simulink model "motor_ctrl_reference"  (R2020b)
settings: Solver=VariableStepAuto  StartTime=0.0  StopTime=1  RelTol=1e-3
InitFcn:
  | Rs=0.43;
  | 
  | Lls=0.002
  | 
  | Rr=0.816;
  | 
  | Llr=0.002
  | 
  | Lm=0.6931;
  | 
  | 
  | J=0.085;
  | np=2;
  | 
  | Ts=1e-5;
  | 
  | Udc=400*sqrt(3)
  | Tpwm = 1e-4;
  | 
  | 
  | 
  | Ls = 1.5*Lm+Lls
  | Lr = 1.5*Lm+Llr
  | Tr = Lr/Rr;
  | sigma = (Ls*Lr-Lm*Lm)/Ls/Lr;
libraries: powerlib x12, simulink x2
settings Model: Creator=messer  LastModifiedBy=messer

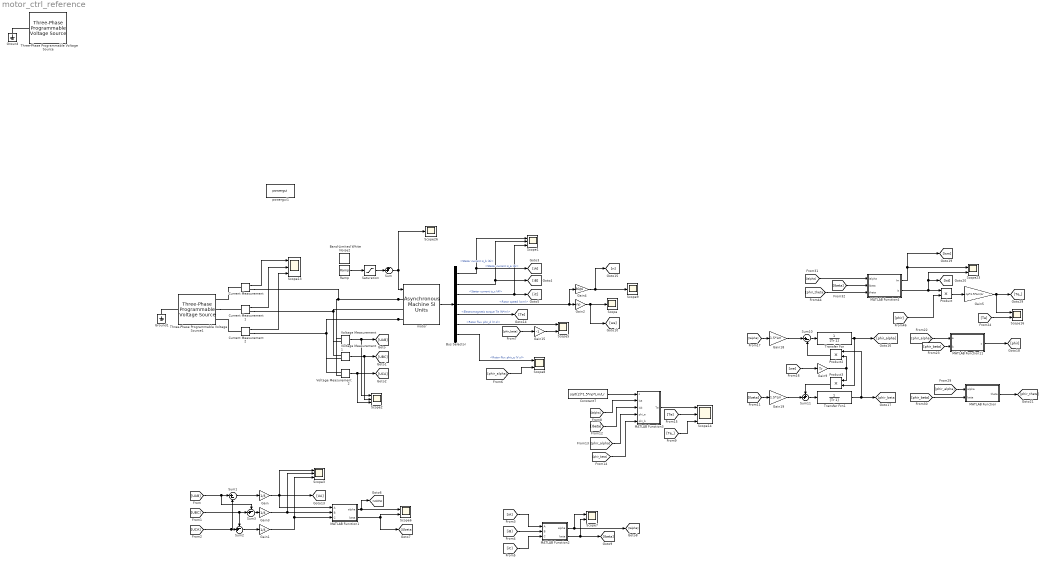
== system motor_ctrl_reference ==
  Band-Limited White Noise2 : simulink/Sources/Band-Limited White Noise  Cov=[0.0001]  Ts=1e-4  seed=[130341]
  Bus Selector : BusSelector  OutputSignals=Stator measurements.Stator current is_a (A),Stator measurements.Stator current is_b (A),Stator measurements.Stator current is_c (A),Mechanical.Rotor speed (wm),Mechanical.Electromagnetic torque Te (N*m),Rotor measurements.Rotor flux phir_d (V s),Rotor measurements.Rotor flux phir_q (V s)
  Constant7 : Constant  Value=sqrt(2)*1.5*np*Lm/Lr
  Current Measurement : powerlib/Measurements/Current Measurement  PhasorSimulation=off  OutputType=Complex  PSBequivalent=0
  Current Measurement1 : powerlib/Measurements/Current Measurement  PhasorSimulation=off  OutputType=Complex  PSBequivalent=0
  Current Measurement2 : powerlib/Measurements/Current Measurement  PhasorSimulation=off  OutputType=Complex  PSBequivalent=0
  Gain : Gain  Gain=1/3
  Gain1 : Gain  Gain=1/3
  Gain15 : Gain  Gain=-1
  Gain18 : Gain  Gain=1.5*Lm
  Gain19 : Gain  Gain=1.5*Lm
  Gain2 : Gain  Gain=np
  Gain3 : Gain  Gain=1/3
  Gain4 : Gain  Gain=30/pi
  Gain5 : Gain  Gain=np*1.5*Lm/Lr
  Gain9 : Gain  Gain=Tr
  Ground : powerlib/Elements/Ground  LConnTagsString=a
  Ground1 : powerlib/Elements/Ground  LConnTagsString=a
  MATLAB Function : MATLAB Function  TreatAsAtomicUnit=on
  MATLAB Function1 : MATLAB Function  TreatAsAtomicUnit=on
  MATLAB Function11 : MATLAB Function  TreatAsAtomicUnit=on
  MATLAB Function2 : MATLAB Function  TreatAsAtomicUnit=on
  MATLAB Function3 : MATLAB Function  TreatAsAtomicUnit=on
  MATLAB Function4 : MATLAB Function  TreatAsAtomicUnit=on
  Product : Product
  Product2 : Product
  Product3 : Product
  Ramp : simulink/Sources/Ramp  slope=100  start=0.25  InitialOutput=5
  Saturation : Saturate  UpperLimit=20  LowerLimit=0
  Scope : Scope
  Scope{1..3,13..14} (5 alike) : Scope  NumInputPorts=3
  Scope{5..8,16,23} (6 alike) : Scope  NumInputPorts=2
  Scope26 : Scope
  Scope9 : Scope
  Sum : Sum  Inputs=++|
  Sum1 : Sum  Inputs=|+-
  Sum10 : Sum  Inputs=|+-
  Sum11 : Sum  Inputs=++|
  Sum2 : Sum  Inputs=-+|
  Sum3 : Sum  Inputs=-+|
  Three-Phase Programmable Voltage Source : powerlib/Electrical Sources/Three-Phase Programmable Voltage Source  PositiveSequence="[380/sqrt(2)  0 50]"  VariationEntity=None  VariationType=Table of time-amplitude pairs  VariationTypeAlt=Step  VariationStep=0.5  VariationRate=10  VariationMagnitude=0.3  VariationFrequency=2  VariationTiming=[1 2]  VariationPhaseA=off  Amplitudes=[1 0.8 1.2 1.0]  TimeValues=[0 0.1 0.15 0.2]  HarmonicGeneration=off  HarmonicA=[3 0.2 -25 0]  HarmonicB=[2 0.15 35 2]  Timing="[0.05  3]"  BusType=swing  Pref=0  Qref=0  Qmin=-inf  Qmax=inf
  Three-Phase Programmable Voltage Source1 : powerlib/Electrical Sources/Three-Phase Programmable Voltage Source  PositiveSequence="[400*sqrt(3/2)  0 120]"  VariationEntity=None  VariationType=Table of time-amplitude pairs  VariationTypeAlt=Step  VariationStep=0.5  VariationRate=10  VariationMagnitude=0.3  VariationFrequency=2  VariationTiming=[1 2]  VariationPhaseA=off  Amplitudes=[1 0.8 1.2 1.0]  TimeValues=[0 0.1 0.15 0.2]  HarmonicGeneration=off  HarmonicA=[3 0.2 -25 0]  HarmonicB=[2 0.15 35 2]  Timing="[0.05  3]"  BusType=swing  Pref=0  Qref=0  Qmin=-inf  Qmax=inf
  Transfer Fcn : TransferFcn  Denominator=[Tr 1]
  Transfer Fcn1 : TransferFcn  Denominator=[Tr 1]
  Voltage Measurement : powerlib/Measurements/Voltage Measurement  PhasorSimulation=off  OutputType=Complex  PSBequivalent=0
  Voltage Measurement1 : powerlib/Measurements/Voltage Measurement  PhasorSimulation=off  OutputType=Complex  PSBequivalent=0
  Voltage Measurement2 : powerlib/Measurements/Voltage Measurement  PhasorSimulation=off  OutputType=Complex  PSBequivalent=0
  motor : powerlib/Machines/Asynchronous Machine SI Units  RotorType=Squirrel-cage  PresetModel=No  MechanicalLoad=Torque Tm  ShowDetailedParameters=on  ReferenceFrame=Stationary  Units=SI  MeasurementBus=off  NominalParameters=[562000 2750 135]  Stator=[Rs Lls]  Rotor=[Rr Llr]  Cage1=[0.4155 0.002066]  Cage2=[0.4168 0.0003495]  Lm=Lm  Mechanical=[J 0 np]  PolePairs=2  InitialConditions=[1 0 0 0 0 0 0 0]  SimulateSaturation=off  Saturation=[14.03593122, 27.81365428, 53.79336849, 72.68890987, 97.98006896, 148.6815601, 215.7428561, 302.9841135, 428.7778367 ; 230, 322, 414, 460, 506, 552, 598, 644, 690]  LoadFlowParameters=1492000  TsPowergui=0  TsBlock=-1  IterativeModel=Trapezoidal non iterative  IterativeDiscreteModel=Trapezoidal non iterative  Pmec=1.492e+006
  powergui1 : powerlib/powergui  Priority=1  SimulationMode=Discrete  SampleTime=2e-6  frequency=60  Iterations=50  frequencyindice=120  Pbase=100e6  ErrMax=1e-4  UnitsV=kV  UnitsW=MW  buscounter=0  FunctionMessages=off  echomessages=off  EnableUseOfTLC=off  CurrentSourceSwitches=off  DisableSnubberDevices=off  DisableRonSwitches=off  DisableVfSwitches=off  DisplayEquations=off  AutomaticDiscreteSolvers=off  SolverType=Tustin/Backward Euler (TBE)  Interpol=off  ExternalGateDelay=off  methode=off  Ts=100  x0status=blocks  SPID=on  SwTol=0  HookPort=off  NonlinearTolerance=1e-4  nMaxIteration=100  ContinueOnMaxIteration=off  RestoreLinks=warning  ResistiveCurrentMeasurement=off  Frange=[0:2:500]  Ylog=off  Xlog=on  ShowGrid=off  save=off  variable=ZData  structure=0  ZoomFFT=off  StartTime=0.0  cycles=1  DisplayStyle=1  fundamental=60  FreqAxis=off  MaxFrequency=1000  frequencyindicesteady=1  RmsSteady=1  display=off
  wires:
  Transfer Fcn/1 -> Product3/2, [phir_alpha]
  Sum10/1 -> Transfer Fcn/1
  MATLAB Function/1(theta) -> [phir_theta]
  Gain9/1 -> Product3/1, Product2/2
  Transfer Fcn1/1 -> Product2/1, [phir_beta]
  Sum11/1 -> Transfer Fcn1/1
  [Ialpha] -> Gain18/1
  [UBC] -> Sum2/1, Sum3/2
  [Ibeta] -> Gain19/1
  Product3/1 -> Sum11/1
  Product2/1 -> Sum10/2
  Gain1/1 -> MATLAB Function1/3(C), Scope3/3
  Gain19/1 -> Sum11/2
  motor/1 -> Bus Selector/1
  MATLAB Function4/1(Im) -> [Ism], Scope23/1
  MATLAB Function11/1(y) -> [phir]
  [we] -> Gain9/1
  [iB] -> MATLAB Function2/2(B)
  Product/1 -> Gain5/1
  [phir_beta] -> MATLAB Function3/5(phi_b)
  [phir_beta] -> MATLAB Function/2(beta)
  Gain18/1 -> Sum10/1
  [phir_theta] -> MATLAB Function4/3(theta)
  MATLAB Function1/2(beta) -> [Ubeta], Scope6/2
  [phir] -> Product/2
  Gain2/1 -> [we], Scope/1
  [Te] -> Scope16/2
  Bus Selector/5 -> [Te]  "<Electromagnetic torque Te (N*m)>"
  [phir_beta] -> Gain15/1
  Gain15/1 -> Scope5/2
  [phir_alpha] -> Scope8/2
  [iA] -> MATLAB Function2/1(A)
  Gain5/1 -> [Te_], Scope16/1
  Current Measurement2/1 -> Scope13/3
  Bus Selector/4 -> Gain4/1, Gain2/1  "<Rotor speed (wm)>"
  [UCA] -> Sum1/2, Sum2/2
  Ramp/1 -> Saturation/1
  Current Measurement1/1 -> Scope13/2
  MATLAB Function2/1(alpha) -> Scope7/1, [Ialpha]
  [Ialpha] -> MATLAB Function4/1(Ialpha)
  Current Measurement/1 -> Scope13/1
  MATLAB Function4/2(It) -> Scope23/2, [Ist], Product/1
  [Ibeta] -> MATLAB Function4/2(Ibeta)
  [phir_beta] -> MATLAB Function11/2(b)
  [phir_alpha] -> MATLAB Function11/1(a)
  MATLAB Function3/1(Te) -> Scope14/1
  Bus Selector/1 -> [iA], Scope1/1  "<Stator current is_a (A)>"
  [phir_alpha] -> MATLAB Function3/4(phi_a)
  Sum/1 -> Scope26/1, motor/1
  Voltage Measurement2/1 -> [UCA], Scope2/3
  Bus Selector/3 -> Scope1/3, [iC]  "<Stator current is_c (A)>"
  Bus Selector/6 -> Scope5/1  "<Rotor flux phir_d (V s)>"
  Gain4/1 -> [n], Scope9/1
  Gain/1 -> MATLAB Function1/1(A), [UA], Scope3/1
  Constant7/1 -> MATLAB Function3/1(c)
  MATLAB Function2/2(beta) -> [Ibeta], Scope7/2
  MATLAB Function1/1(alpha) -> [Ualpha], Scope6/1
  [phir_alpha] -> MATLAB Function/1(alpha)
  [Ialpha] -> MATLAB Function3/2(isa)
  [UAB] -> Sum3/1, Sum1/1
  [Te_] -> Scope14/3
  [Te] -> Scope14/2
  Bus Selector/2 -> Scope1/2, [iB]  "<Stator current is_b (A)>"
  [Ibeta] -> MATLAB Function3/3(isb)
  Sum3/1 -> Gain3/1
  Sum1/1 -> Gain/1
  [iC] -> MATLAB Function2/3(C)
  Saturation/1 -> Sum/2
  Voltage Measurement1/1 -> [UBC], Scope2/2
  Sum2/1 -> Gain1/1
  Bus Selector/7 -> Scope8/1  "<Rotor flux phir_q (V s)>"
  Gain3/1 -> MATLAB Function1/2(B), Scope3/2
  Voltage Measurement/1 -> Scope2/1, [UAB]
  connections:
  Ground/LConn1 -- Three-Phase Programmable Voltage Source/LConn1
  motor/LConn1 -- Voltage Measurement/LConn1 -- Voltage Measurement2/LConn2 -- Current Measurement/RConn1
  Current Measurement1/RConn1 -- Voltage Measurement1/LConn1 -- Voltage Measurement/LConn2 -- motor/LConn2
  motor/LConn3 -- Current Measurement2/RConn1 -- Voltage Measurement2/LConn1 -- Voltage Measurement1/LConn2
  Ground1/LConn1 -- Three-Phase Programmable Voltage Source1/LConn1
  Three-Phase Programmable Voltage Source1/RConn2 -- Current Measurement1/LConn1
  Current Measurement/LConn1 -- Three-Phase Programmable Voltage Source1/RConn1
  Current Measurement2/LConn1 -- Three-Phase Programmable Voltage Source1/RConn3

== matlab function motor_ctrl_reference/MATLAB Function1 ==
  data: A input; alpha output; B input; C input; beta output
function [alpha, beta] = fcn(A, B, C)
k = 2/ 3;
alpha = k * (A - 0.5*B - 0.5*C);
beta = k * sqrt(3) / 2 * (B - C);

== matlab function motor_ctrl_reference/MATLAB Function2 ==
  data: A input; alpha output; B input; C input; beta output
function [alpha, beta] = fcn(A, B, C)
k = 2/ 3;
alpha = k * (A - 0.5*B - 0.5*C);
beta = k * sqrt(3) / 2 * (B - C);

== matlab function motor_ctrl_reference/MATLAB Function3 ==
  data: c input; Te output; isa input; isb input; phi_a input; phi_b input
function Te = fcn(c, isa, isb, phi_a, phi_b)
Te = c *( isb * phi_a - isa * phi_b);

== matlab function motor_ctrl_reference/MATLAB Function4 ==
  data: Im output; Ialpha input; Ibeta input; theta input; It output
function [Im, It] = fcn(Ialpha, Ibeta, theta)

Im = Ialpha * cos(theta) + Ibeta * sin(theta);
It = -Ialpha * sin(theta) + Ibeta * cos(theta);

== matlab function motor_ctrl_reference/MATLAB Function11 ==
  data: y output; a input; b input
function y = fcn(a, b)

y = sqrt(a*a + b*b);

== matlab function motor_ctrl_reference/MATLAB Function ==
  data: theta output; alpha input; beta input
function theta = fcn(alpha, beta)

if(beta >=0)
    if(alpha == 0)
        theta = pi/2;
    elseif(alpha >0)
        theta = atan(beta/alpha);
    else
        theta = pi + atan(beta/alpha);
    end
else
    if(alpha == 0)
        theta = 1.5*pi;
    elseif(alpha > 0)
        theta = 2*pi + atan(beta/alpha);
    else
        theta = pi + atan(beta/alpha);
    end
end
